simulink model "untitled1"  (R2016a)
settings: Solver=FixedStepAuto  StartTime=0.0  StopTime=2.38  FixedStep=0.001  RelTol=1e-3
undefined symbols (not defined in the file): data, init, Ts, w, wn
settings Model: Creator=hqm3yy  LastModifiedBy=hqm3yy
settings GRTTargetCC: GeneratePreprocessorConditionals=Use local settings

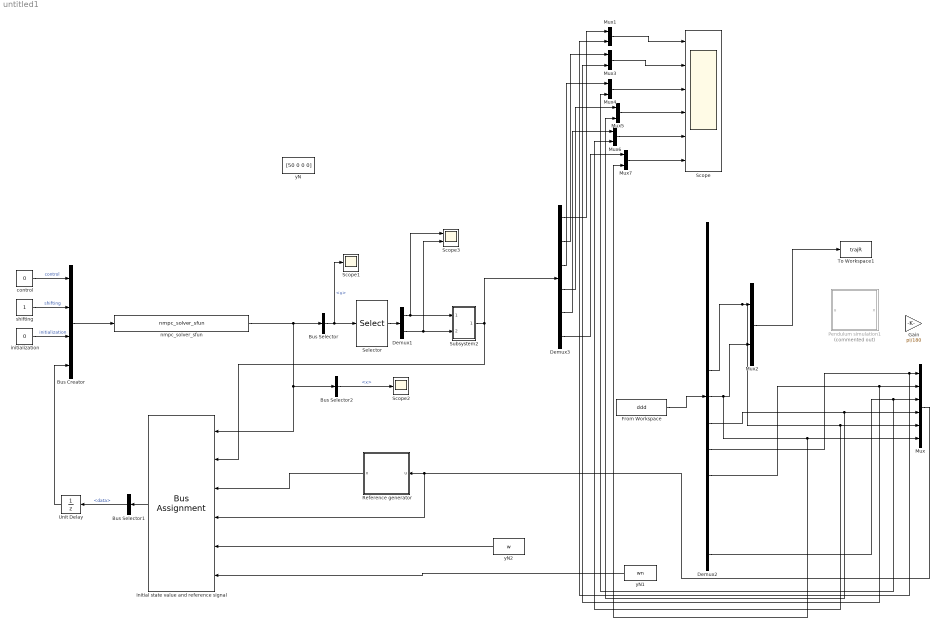
== system untitled1 ==
  Bus Creator : BusCreator  Inputs=4  OutDataTypeStr=Bus: ACADOinput
  Bus Selector : BusSelector  OutputSignals=data.u
  Bus Selector1 : BusSelector  OutputSignals=data
  Bus Selector2 : BusSelector  OutputSignals=data.x
  Demux1 : Demux  Outputs=2
  Demux2 : Demux  Outputs=13
  Demux3 : Demux  Outputs=6
  From Workspace : FromWorkspace  VariableName=ddd  SampleTime=0.001
  Gain : Gain  Gain=pi/180
  Initial state value and reference signal : BusAssignment  AssignedSignals=data.x0,data.y,data.yN,data.W,data.WN
  Mux : Mux  Inputs=6
  Mux{1..7} (7 alike) : Mux  Inputs=2
  Pendulum simulation1 : Subsystem  Commented=on
      mask help: Simple system simulation.
      mask init:
      | % initialize state values
      mask Display: disp('System');
  Reference generator : Subsystem
      mask help: Simple system simulation.
      mask init:
      | % initialize state values
      mask Display: disp('System');
  Scope : Scope  NumInputPorts=6
  Scope1 : Scope
  Scope2 : Scope
  Scope3 : Scope  NumInputPorts=2
  Selector : Selector  InputPortWidth=160  IndexOptions=Index vector (dialog)  Indices=[1 2]  OutputSizes=2
  Subsystem2 : Subsystem
  To Workspace1 : ToWorkspace  VariableName=trajR  SampleTime=-1
  Unit Delay : UnitDelay  InitialCondition=init  SampleTime=Ts
  control : Constant  Value=0  OutDataTypeStr=int32
  initialization : Constant  Value=0  OutDataTypeStr=int32
  nmpc_solver_sfun : S-Function  FunctionName=nmpc_solver_sfun  SFunctionDeploymentMode=off  EnableBusSupport=off  mask(Legacy Function){SFunctionSpec=nmpc_step(ACADOinput u1[1], ACADOoutput y1[1]), ShowSpec=on}
      mask prompts: ShowSpec "Display function specification"
      mask help:
      | This block allows you to call the legacy functions specified by the following Legacy Code Tool definition:
      | def.SFunctionName = 'nmpc_solver_sfun';
      | def.OutputFcnSpec = 'nmpc_step(ACADOinput u1[1], ACADOoutput y1[1])';
      | def.StartFcnSpec = 'nmpc_initialize( void )';
      | def.TerminateFcnSpec = 'nmpc_cleanup( void )';
      | def.HeaderFiles = {'nmpc_common.h', 'nmpc_solver_sfunction.h'};
      | def.SourceFiles = {'nmpc_solver.c', 'nmpc_integrator.c', 'nmpc_auxiliary_functions.c', 'nmpc_solver_sfunction.c', 'nmpc_qpoases_interface.cpp', 'qpoases\SRC\Bounds.cpp', 'qpoases\SRC\Constraints.cpp', 'qpoases\SRC\CyclingManager.cpp', 'qpoases\SRC\Indexlist.cpp', 'qpoases\SRC\MessageHandling.cpp', 'qpoases\SRC\QProblem.cpp', 'qpoases\SRC\QProblemB.cpp', 'qpoases\SRC\SubjectTo.cpp', 'qpoases\SRC\Utils.cpp', 'qpoases\SRC\EXTRAS\SolutionAnalysis.cpp'};
      | def.IncPaths = {'qpoases', 'qpoases/INCLUDE', 'qpoases/SRC'};
      | def.Options.language = 'C++';
      mask Help: <p>This block was generated automatically by the Legacy Code Tool. For detailed help on this tool, call<a href="matlab:legacy_code('help')"> legacy_code('help')</a>.</p>
      mask Callback ShowSpec:
      | if strcmp(get_param(gcbh, 'ShowSpec'), 'on')
      |   set_param(gcbh, 'MaskDisplay', sprintf('fprintf(''%s'');', get_param(gcbh, 'SFunctionSpec')));
      | else
      |   set_param(gcbh, 'MaskDisplay', sprintf('fprintf(''%s'');', get_param(gcbh, 'FunctionName')));
      | end
      mask Display: fprintf('nmpc_step(ACADOinput u1[1], ACADOoutput y1[1])');
  shifting : Constant  OutDataTypeStr=int32
  yN : Constant  Value=[50 0 0 0]  OutDataTypeStr=double
  yN1 : Constant  Value=wn  OutDataTypeStr=double
  yN2 : Constant  Value=w  OutDataTypeStr=double
  wires:
  Initial state value and reference signal/1 -> Bus Selector1/1
  Bus Selector/1 -> Selector/1, Scope1/1  "<u>"
  Selector/1 -> Demux1/1
  Bus Selector1/1 -> Unit Delay/1  "<data>"
  Unit Delay/1 -> Bus Creator/4
  shifting/1 -> Bus Creator/2  "shifting"
  control/1 -> Bus Creator/1  "control"
  initialization/1 -> Bus Creator/3  "initialization"
  yN2/1 -> Initial state value and reference signal/5
  yN1/1 -> Initial state value and reference signal/6
  Bus Selector2/1 -> Scope2/1  "<x>"
  From Workspace/1 -> Demux2/1
  Demux2/6 -> Mux6/2, Mux/5, Mux2/1
  Mux2/1 -> To Workspace1/1
  Demux1/2 -> Scope3/2, Subsystem2/2(Acceleration U2)
  Demux1/1 -> Scope3/1, Subsystem2/1(Steering U1)
  Demux2/9 -> Mux1/2, Mux/1
  Demux2/10 -> Mux3/2, Mux/2
  Demux2/13 -> Mux4/2, Mux/3
  Demux2/8 -> Mux5/2, Mux/4
  Demux2/7 -> Mux7/2, Mux/6, Mux2/2
  Mux/1 -> Reference generator/1(u), Initial state value and reference signal/4
  Bus Creator/1 -> nmpc_solver_sfun/1
  nmpc_solver_sfun/1 -> Initial state value and reference signal/1, Bus Selector2/1, Bus Selector/1
  Subsystem2/1(Out1) -> Initial state value and reference signal/2, Demux3/1
  Mux1/1 -> Scope/1
  Demux3/1 -> Mux1/1
  Mux3/1 -> Scope/2
  Demux3/2 -> Mux3/1
  Mux4/1 -> Scope/3
  Demux3/3 -> Mux4/1
  Mux5/1 -> Scope/4
  Demux3/4 -> Mux5/1
  Mux6/1 -> Scope/5
  Demux3/5 -> Mux6/1
  Mux7/1 -> Scope/6
  Demux3/6 -> Mux7/1
  Reference generator/1(x) -> Initial state value and reference signal/3

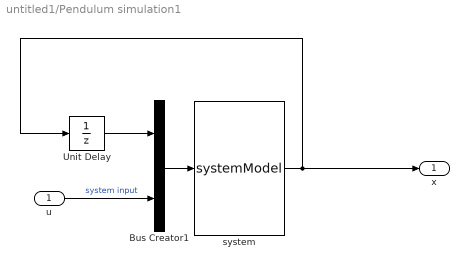
== system untitled1/Pendulum simulation1 ==
  u : Inport
  Bus Creator1 : BusCreator  Inputs=2
  Unit Delay : UnitDelay  InitialCondition=init.x0  SampleTime=Ts
  system : S-Function  FunctionName=systemModel  SFunctionDeploymentMode=off  EnableBusSupport=off
  x : Outport
  wires:
  u/1 -> Bus Creator1/2  "system input"
  Bus Creator1/1 -> system/1
  system/1 -> x/1, Unit Delay/1
  Unit Delay/1 -> Bus Creator1/1

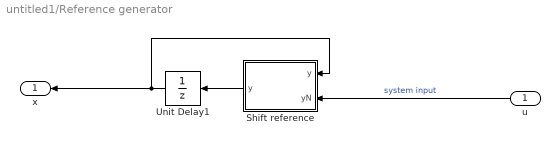
== system untitled1/Reference generator ==
  u : Inport
  Shift reference : MATLAB Function  TreatAsAtomicUnit=on
  Unit Delay1 : UnitDelay  InitialCondition=init.y  SampleTime=Ts
  x : Outport
  wires:
  u/1 -> Shift reference/2(yN)  "system input"
  Shift reference/1(y) -> Unit Delay1/1
  Unit Delay1/1 -> x/1, Shift reference/1("y ")

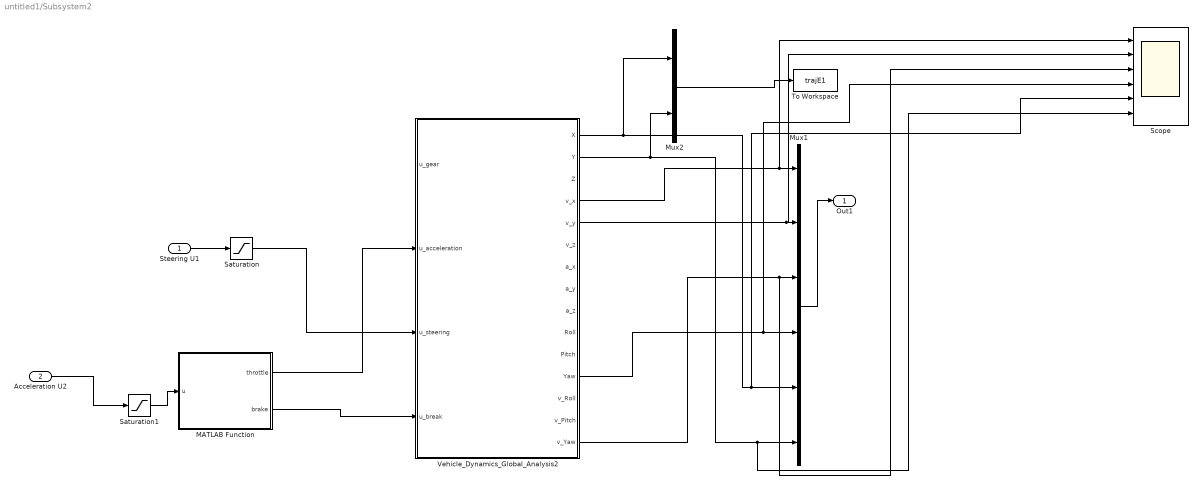
== system untitled1/Subsystem2 ==
  Steering U1 : Inport
  Acceleration U2 : Inport  Port=2
  MATLAB Function : MATLAB Function  TreatAsAtomicUnit=on
  Mux1 : Mux  Inputs=6
  Mux2 : Mux  Inputs=2
  Saturation : Saturate  UpperLimit=1  LowerLimit=-1
  Saturation1 : Saturate  UpperLimit=1  LowerLimit=-1
  Scope : Scope  NumInputPorts=6
  To Workspace : ToWorkspace  VariableName=trajE1  SampleTime=-1
  Vehicle_Dynamics_Global_Analysis2 : Subsystem  Tag=AME2SLCoSim  InitFcn=AMESimLib_initBlock  StartFcn=AMESimLib_startBlock  StopFcn=AMESimLib_stopBlock
      settings: DeleteFcn=AMESimLib_deleteBlock  OpenFcn=AMESimLib_openBlock('AME2SLCoSim')
      mask Display: image(imread('amesim_pix256.png'),[0.4,0.7,0.2,0.2]);disp('Simcenter Amesim co-Sim:\nVehicle_Dynamics_Global_Analysis2');port_label('input',1,'u_gear');port_label('input',2,'u_acceleration');port_label('input',3,'u_steering');port_label('input',4,'u_break');port_label('output',1,'X');port_label('output',2,'Y');port_label('output',3,'Z');port_label('output',4,'v_x');port_label('output',5,'v_y');port_label('output',6,'v_z');port_label('output',7,'a_x');port_label('output',8,'a_y');port_label('output',9,'a_z');port_label('output',10,'Roll');port_label('output',11,'Pitch');port_label('output',12,'Yaw');port_label('output',13,'v_Roll');port_label('output',14,'v_Pitch');port_label('output',15,'v_Yaw');
  Out1 : Outport
  wires:
  Mux1/1 -> Out1/1
  Acceleration U2/1 -> Saturation1/1
  MATLAB Function/1(throttle) -> Vehicle_Dynamics_Global_Analysis2/2(u_acceleration)
  MATLAB Function/2(brake) -> Vehicle_Dynamics_Global_Analysis2/4(u_break)
  Steering U1/1 -> Saturation/1
  Vehicle_Dynamics_Global_Analysis2/4(v_x) -> Scope/1, Mux1/1
  Vehicle_Dynamics_Global_Analysis2/5(v_y) -> Scope/2, Mux1/2
  Vehicle_Dynamics_Global_Analysis2/15(v_Yaw) -> Scope/3, Mux1/3
  Vehicle_Dynamics_Global_Analysis2/12(Yaw) -> Scope/4, Mux1/4
  Vehicle_Dynamics_Global_Analysis2/1(X) -> Mux2/1, Scope/5, Mux1/5
  Vehicle_Dynamics_Global_Analysis2/2(Y) -> Mux2/2, Scope/6, Mux1/6
  Mux2/1 -> To Workspace/1
  Saturation/1 -> Vehicle_Dynamics_Global_Analysis2/3(u_steering)
  Saturation1/1 -> MATLAB Function/1(u)

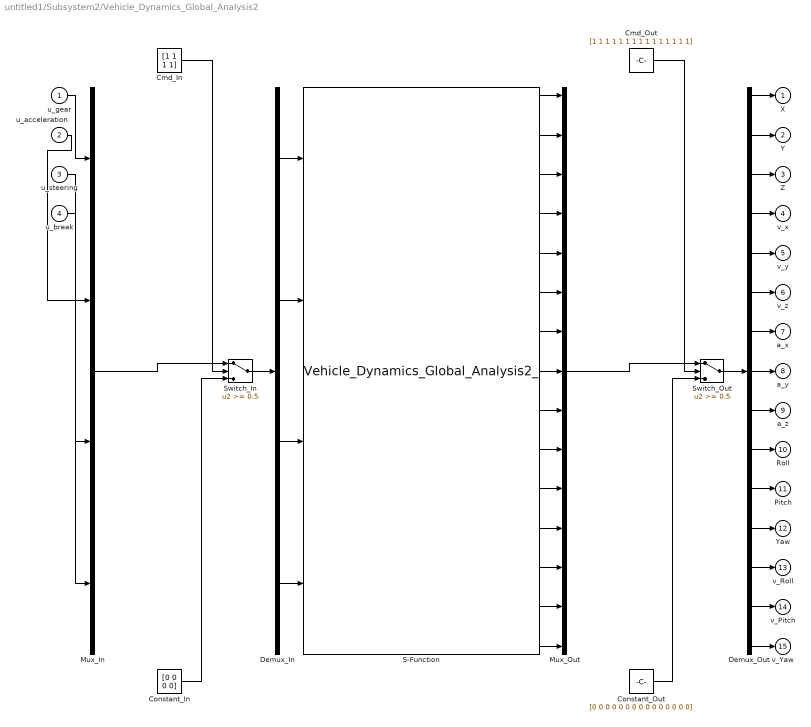
== system untitled1/Subsystem2/Vehicle_Dynamics_Global_Analysis2 ==
  u_gear : Inport
  u_acceleration : Inport  Port=2
  u_steering : Inport  Port=3
  u_break : Inport  Port=4
  Cmd_In : Constant  Value=[1 1 1 1]
  Cmd_Out : Constant  Value=[1 1 1 1 1 1 1 1 1 1 1 1 1 1 1]
  Constant_In : Constant  Value=[0 0 0 0]
  Constant_Out : Constant  Value=[0 0 0 0 0 0 0 0 0 0 0 0 0 0 0]
  Demux_In : Demux
  Demux_Out : Demux  Outputs=15
  Mux_In : Mux
  Mux_Out : Mux  Inputs=15
  S-Function : S-Function  InitFcn=clear Vehicle_Dynamics_Global_Analysis2_  StopFcn=clear Vehicle_Dynamics_Global_Analysis2_  FunctionName=Vehicle_Dynamics_Global_Analysis2_  Parameters="[0.001;0.001;1e-05;1e+30;100;0;0;2;0;1;0.001;0;1] ['Grav           ';'Xg             ';'Zg             ';'V0             ';'Msprung        ';'Msteer         ';'Msp_front      ';'Mwh_front      ';'Msp_rear       ';'Mwh_rear       ';'Isprung_xx     ';'Isprung_yy     ';'Isprung_zz     ';'Isprung_xy     ';'Isprung_xz     ';'Isprung_yz     ';'Zref_front     ';'Zref_rear      ';'wheelbase      ';'track_front    ';'track_rear     ';'Rpinion        ';'Ksusp_front    ';'Ksusp_rear     ';'Rsusp_front    ';'Rsusp_rear     ';'Kantiroll_front';'Kantiroll_rear ';'Rfree          ';'Rroll          ';'Ktire          ';'Rtire          ';'a1             ';'a2             ';'a3             ';'a4             '] [9.8066;1056;375;0;1300;2;18;18;15;14;250;1000;1300;0;-20;0;75;75;2400;1450;1450;8;21000;21000;2000;1500;30000;20000;0.292;0.29;200000;100;-50;1200;1000;5] [] [] [] []"  SFunctionDeploymentMode=off  EnableBusSupport=off
      mask Display: port_label('output',1,'X');port_label('output',2,'Y');port_label('output',3,'Z');port_label('output',4,'v_x');port_label('output',5,'v_y');port_label('output',6,'v_z');port_label('output',7,'a_x');port_label('output',8,'a_y');port_label('output',9,'a_z');port_label('output',10,'Roll');port_label('output',11,'Pitch');port_label('output',12,'Yaw');port_label('output',13,'v_Roll');port_label('output',14,'v_Pitch');port_label('output',15,'v_Yaw');port_label('input',1,'u_gear');port_label('input',2,'u_acceleration');port_label('input',3,'u_steering');port_label('input',4,'u_break');disp('Simcenter Amesim:\n Vehicle_Dynamics_Global_Analysis2_')
  Switch_In : Switch  Threshold=0.5  SaturateOnIntegerOverflow=on  InputSameDT=on
  Switch_Out : Switch  Threshold=0.5  SaturateOnIntegerOverflow=on  InputSameDT=on
  X : Outport
  Y : Outport  Port=2
  Z : Outport  Port=3
  v_x : Outport  Port=4
  v_y : Outport  Port=5
  v_z : Outport  Port=6
  a_x : Outport  Port=7
  a_y : Outport  Port=8
  a_z : Outport  Port=9
  Roll : Outport  Port=10
  Pitch : Outport  Port=11
  Yaw : Outport  Port=12
  v_Roll : Outport  Port=13
  v_Pitch : Outport  Port=14
  v_Yaw : Outport  Port=15
  wires:
  Mux_In/1 -> Switch_In/1
  Cmd_In/1 -> Switch_In/2
  Constant_In/1 -> Switch_In/3
  Switch_In/1 -> Demux_In/1
  Mux_Out/1 -> Switch_Out/1
  Cmd_Out/1 -> Switch_Out/2
  Constant_Out/1 -> Switch_Out/3
  Switch_Out/1 -> Demux_Out/1
  u_gear/1 -> Mux_In/1
  Demux_In/1 -> S-Function/1
  u_acceleration/1 -> Mux_In/2
  Demux_In/2 -> S-Function/2
  u_steering/1 -> Mux_In/3
  Demux_In/3 -> S-Function/3
  u_break/1 -> Mux_In/4
  Demux_In/4 -> S-Function/4
  Demux_Out/1 -> X/1
  S-Function/1 -> Mux_Out/1
  Demux_Out/2 -> Y/1
  S-Function/2 -> Mux_Out/2
  Demux_Out/3 -> Z/1
  S-Function/3 -> Mux_Out/3
  Demux_Out/4 -> v_x/1
  S-Function/4 -> Mux_Out/4
  Demux_Out/5 -> v_y/1
  S-Function/5 -> Mux_Out/5
  Demux_Out/6 -> v_z/1
  S-Function/6 -> Mux_Out/6
  Demux_Out/7 -> a_x/1
  S-Function/7 -> Mux_Out/7
  Demux_Out/8 -> a_y/1
  S-Function/8 -> Mux_Out/8
  Demux_Out/9 -> a_z/1
  S-Function/9 -> Mux_Out/9
  Demux_Out/10 -> Roll/1
  S-Function/10 -> Mux_Out/10
  Demux_Out/11 -> Pitch/1
  S-Function/11 -> Mux_Out/11
  Demux_Out/12 -> Yaw/1
  S-Function/12 -> Mux_Out/12
  Demux_Out/13 -> v_Roll/1
  S-Function/13 -> Mux_Out/13
  Demux_Out/14 -> v_Pitch/1
  S-Function/14 -> Mux_Out/14
  Demux_Out/15 -> v_Yaw/1
  S-Function/15 -> Mux_Out/15

== matlab function untitled1/Subsystem2/MATLAB Function ==
  data: u input; throttle output; brake output
function [throttle, brake]= fcn(u)
%#codegen

if u > 0
    throttle = 1*abs(u);
    brake = 0;
else
    brake = 1*abs(u);
    throttle = 0;
end



end

== matlab function untitled1/Reference generator/Shift reference ==
  data: y input; y output; yN input
function y = shift_reference(y, yN)

NX = 6;
NU = 2;

y = [y(NX+NU+1:end);yN;y(end-NU+1:end)];
